simulink model "Model_of_3DOF_manipulator"  (R2023a)
settings: Solver=VariableStepAuto  StartTime=0.0  StopTime=1  RelTol=1e-3  AbsTol=1e-3
values from neighbouring files (symbols this model uses):
  K1_d = 19.4    [parameters.m]
  K1_I_xx = 9.4    [parameters.m]
  K1_I_yy = 9.4    [parameters.m]
  K1_I_zz = 0.7    [parameters.m]
  K1_K1 = 3880    [parameters.m]
  K1_K2 = 2.94    [parameters.m]
  K1_K3 = 96    [parameters.m]
  K1_K4 = 0.044    [parameters.m]
  K1_K5 = 156    [parameters.m]
  K1_l = 0.7    [parameters.m]
  K1_m = 46    [parameters.m]
  K2_d = 24.7    [parameters.m]
  K2_I_xx = 16.5    [parameters.m]
  K2_I_yy = 16.5    [parameters.m]
  K2_I_zz = 0.7    [parameters.m]
  K2_K1 = 2330    [parameters.m]
  K2_K2 = 2.8    [parameters.m]
  K2_K3 = 117    [parameters.m]
  K2_K4 = 0.043    [parameters.m]
  K2_K5 = 94    [parameters.m]
  K2_l = 0.55    [parameters.m]
  K2_m = 78    [parameters.m]
  P_d = 30.2    [parameters.m]
  P_I_xx = 33.3    [parameters.m]
  P_I_yy = 33.3    [parameters.m]
  P_I_zz = 9.1    [parameters.m]
  P_K1 = 4202    [parameters.m]
  P_K2 = 2.97    [parameters.m]
  P_K3 = 120    [parameters.m]
  P_K4 = 0.055    [parameters.m]
  P_K5 = 168    [parameters.m]
  P_l = 0.875    [parameters.m]
  P_m = 194    [parameters.m]
undefined symbols (not defined in the file or in its folder): X, Y, Z
libraries: sm_lib x21, nesl_utility x17
settings Model: Creator=ПК  LastModifiedBy=ПК
settings SolverCC: AutoScaleAbsTol=off  AlgebraicLoopSolver=TrustRegion  MaxZcPerStep=1
settings DebuggingCC: UnconnectedInputMsg=warning  UnconnectedOutputMsg=warning  UnconnectedLineMsg=warning  SymbolicDimsDataTypeCodeGenerationDiagnostic=none
settings ModelReferenceCC: EnableRefExpFcnMdlSchedulingChecks=on
settings SFSimCC: CustomCodeUndefinedFunction=UseInterfaceOnly
settings RTWCC: DLArmComputeVersion=19.05
settings SimscapeCC: SimscapeLogType=all  SimscapeLogSimulationStatistics=on  SimscapeLogDataHistory=10000

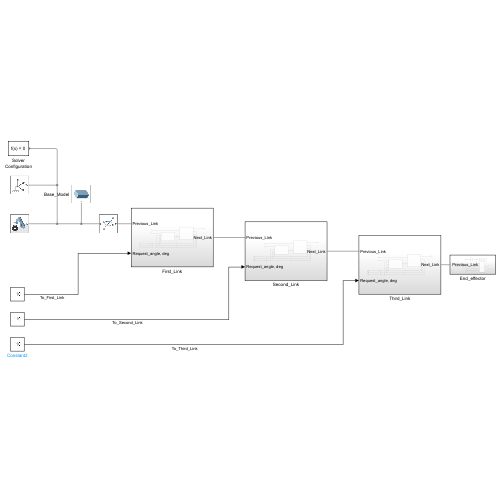
[thumbnail: Simulink's stored preview of the top-level diagram]
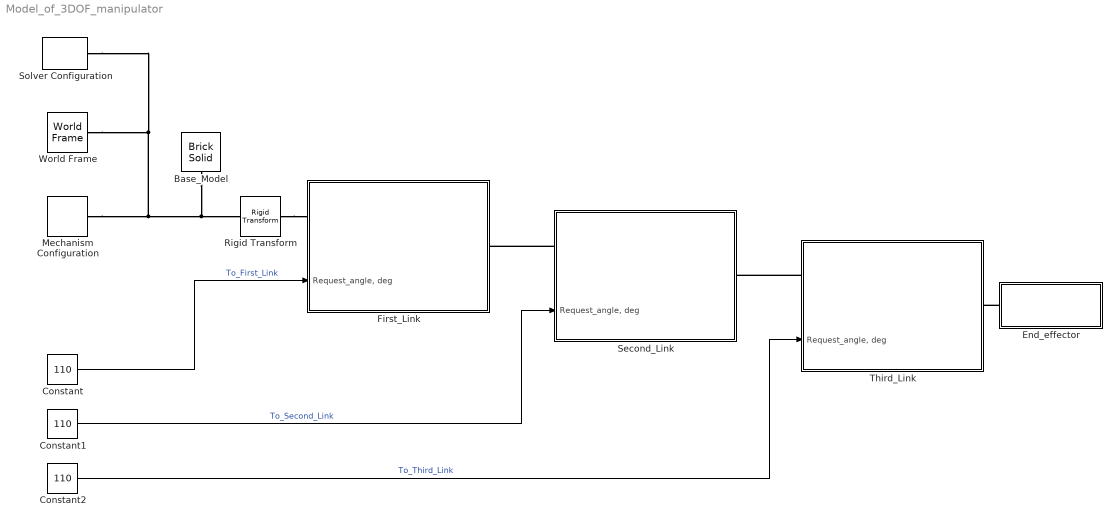
== system Model_of_3DOF_manipulator ==
  Base_Model : sm_lib/Body Elements/Brick Solid  GraphicAmbientColor=[0.15 0.15 0.15 1.0]  BasedOnType=Density  BrickDimensions=[0.5 0.5 0.5]  BrickDimensionsUnits=m  CenterOfMass=[0 0 0]  CenterOfMassUnits=m  GraphicDiffuseColor=[0.5 0.5 0.5]  Density=1000  DensityUnits=kg/m^3  DoExposeReferenceFrame=on  GraphicEmissiveColor=[0.0 0.0 0.0 1.0]  ExportEntireGeometry=off  SerializedFrames=<Frames/>  MarkerShape=Sphere  MarkerSize=10  GraphicType=FromGeometry  InertiaType=CalculateFromGeometry  Mass=1  MassUnits=kg  MomentsOfInertia=[1 1 1]  MomentsOfInertiaUnits=kg*m^2  GraphicOpacity=1.0  ProductsOfInertia=[0 0 0]  ProductsOfInertiaUnits=kg*m^2  GraphicShininess=75  GraphicSpecularColor=[0.5 0.5 0.5 1.0]  GraphicVisPropType=SimpleVisualProperties
  Constant : Constant  Value=110
  Constant1 : Constant  Value=110
  Constant2 : Constant  Value=110
  End_effector : Subsystem
  First_Link : Subsystem
      settings: PortSchema="{\"entries\":[{\"content\":{\"sides\":[{\"content\":{\"connectorIds\":[\"LConn1\",\"In1\"]},\"type\":\"ConnectorPlacement.EquallySpacedRectSide\",\"uuid\":\"66fdbe92-d6ab-4206-84fe-86206e1853da\"},{\"content\":{\"connectorIds\":[\"RConn1\"],\"side\":\"RIGHT\"},\"type\":\"ConnectorPlacement.EquallySpacedRectSide\",\"uuid\":\"85951761-cf01-4a63-8fcb-bb43d3271314\"},{\"content\":{\"side\":\"TOP\"},\"type\":\"ConnectorPlacement.EquallySpacedRectSide\",\"uuid\":\"eebc5883-fa22-4c85-b57d-f4e866a15e11\"}]},\"type\":\"ConnectorPlacement.EquallySpacedConnector\",\"uuid\":\"c98930f2-9c31-48e8-8f38-2652a55b5104\"}],\"packageUris\":[\"http://schema.mathworks.com/mf0/Connector/R2020b\"],\"version\":\"1.0\"}"
  Mechanism Configuration : sm_lib/Utilities/Mechanism Configuration  UniformGravity=Constant  GravityVector=[0 -9.80665 0]  GravityVectorUnits=m/s^2  LinearizationDelta=0.001  JointModeTransitionNonlinearIterations=2
  Rigid Transform : sm_lib/Frames and Transforms/Rigid Transform  TranslationMethod=Cartesian  TranslationStandardOffset=0  TranslationStandardOffsetUnits=m  TranslationStandardAxis=+Z  TranslationCartesianOffset=[0 0 0.25]  TranslationCartesianOffsetUnits=m  TranslationROffset=0  TranslationROffsetUnits=m  TranslationZOffset=0  TranslationZOffsetUnits=m  TranslationThetaOffset=0  TranslationThetaOffsetUnits=deg  RotationMethod=None  RotationAngleUnits=deg  RotationStandardAxis=+Z  RotationAngle=0.0  RotationArbitraryAxis=[0 0 1]  FollAlignAxisA=+X  BaseAlignAxisA=+Y  FollAlignAxisB=+Y  BaseAlignAxisB=+Z  RotationSequenceAxes=FollowerAxes  RotationSequence=XYX  RotationSequenceAngles=[0 0 0]  RotationSequenceAnglesUnits=deg  RotationMatrix=[1 0 0; 0 1 0; 0 0 1]  Quaternion=[1 0 0 0]
  Second_Link : Subsystem
      settings: PortSchema="{\"entries\":[{\"content\":{\"sides\":[{\"content\":{\"connectorIds\":[\"LConn1\",\"In1\"]},\"type\":\"ConnectorPlacement.EquallySpacedRectSide\",\"uuid\":\"66fdbe92-d6ab-4206-84fe-86206e1853da\"},{\"content\":{\"connectorIds\":[\"RConn1\"],\"side\":\"RIGHT\"},\"type\":\"ConnectorPlacement.EquallySpacedRectSide\",\"uuid\":\"85951761-cf01-4a63-8fcb-bb43d3271314\"},{\"content\":{\"side\":\"TOP\"},\"type\":\"ConnectorPlacement.EquallySpacedRectSide\",\"uuid\":\"eebc5883-fa22-4c85-b57d-f4e866a15e11\"}]},\"type\":\"ConnectorPlacement.EquallySpacedConnector\",\"uuid\":\"c98930f2-9c31-48e8-8f38-2652a55b5104\"}],\"packageUris\":[\"http://schema.mathworks.com/mf0/Connector/R2020b\"],\"version\":\"1.0\"}"
  Solver Configuration : nesl_utility/Solver Configuration  PhysicalDomain=network_engine_domain  SubClassName=solver  LeftPortType=input  RightPortType=generic  Tones=[]  Harmonics=[]  SimulateNoise=off  Profile=off  UseLocalSampling=off  EnableSwitchedLinearOptims=on  FrequencyDomain=off  UseCCode=off  RelTol=0.001  AbsTol=1e-06  MinStep=1e-09  ToWorkspace=off  RevertToSquareIcSolve=off  NumHomotopyIterations=100  PhasorMode=off  PhasorModeNumHarmonics=1  ConsistencySolver=NEWTON_XTOL_AFTER_FTOL  IndexReductionMethod=DerivativeReplacement  DoDC=off  ResidualTolerance=1e-09  ConsistencyTolSource=GLOBAL  ConsistencyAbsTol=0.001  ConsistencyRelTol=0.001  ConsistencyTolFactor=0.001  UseLocalSolver=off  LocalSolverChoice=NE_BACKWARD_EULER_ADVANCER  ResolveIndetEquations=on  FunctionEvalNumThread=1  LocalSolverSampleTime=0.001  DoFixedCost=off  MaxNonlinIter=3  MaxModeIter=2  ComputeImpulses=off  ImpulseIterations=2  LinearAlgebra=auto  LinearAlgebraNumThread=0  EquationFormulation=NE_TIME_EF  DelaysMemoryBudget=1024  AutomaticFiltering=on  FilteringTimeConstant=0.001  PartitionStorageMethod=AS_NEEDED  PartitionMemoryBudget=1024  PartitionMethod=ROBUST
  Third_Link : Subsystem
      settings: PortSchema="{\"entries\":[{\"content\":{\"sides\":[{\"content\":{\"connectorIds\":[\"LConn1\",\"In1\"]},\"type\":\"ConnectorPlacement.EquallySpacedRectSide\",\"uuid\":\"66fdbe92-d6ab-4206-84fe-86206e1853da\"},{\"content\":{\"connectorIds\":[\"RConn1\"],\"side\":\"RIGHT\"},\"type\":\"ConnectorPlacement.EquallySpacedRectSide\",\"uuid\":\"85951761-cf01-4a63-8fcb-bb43d3271314\"},{\"content\":{\"side\":\"TOP\"},\"type\":\"ConnectorPlacement.EquallySpacedRectSide\",\"uuid\":\"eebc5883-fa22-4c85-b57d-f4e866a15e11\"}]},\"type\":\"ConnectorPlacement.EquallySpacedConnector\",\"uuid\":\"c98930f2-9c31-48e8-8f38-2652a55b5104\"}],\"packageUris\":[\"http://schema.mathworks.com/mf0/Connector/R2020b\"],\"version\":\"1.0\"}"
  World Frame : sm_lib/Frames and Transforms/World Frame
  wires:
  Constant/1 -> First_Link/1("Request_angle, deg")  "To_First_Link"
  Constant1/1 -> Second_Link/1("Request_angle, deg")  "To_Second_Link"
  Constant2/1 -> Third_Link/1("Request_angle, deg")  "To_Third_Link"
  connections:
  Second_Link/LConn1 -- First_Link/RConn1
  World Frame/RConn1 -- Mechanism Configuration/RConn1 -- Rigid Transform/LConn1 -- Base_Model/RConn1 -- Solver Configuration/RConn1
  Third_Link/LConn1 -- Second_Link/RConn1
  Rigid Transform/RConn1 -- First_Link/LConn1
  End_effector/LConn1 -- Third_Link/RConn1

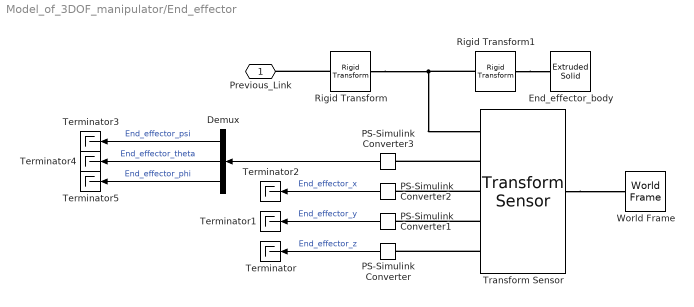
== system Model_of_3DOF_manipulator/End_effector ==
  Demux : Demux  Outputs=3
  End_effector_body : sm_lib/Body Elements/Extruded Solid  GraphicAmbientColor=[0.15 0.15 0.15 1.0]  BasedOnType=Density  CenterOfMass=[0 0 0]  CenterOfMassUnits=m  GraphicDiffuseColor=[0.5 0.5 0.5]  ExportConvexHullGeometry=off  ExtrusionCrossSection=[1 1; -1 1; -1 -1; 1 -1]  ExtrusionCrossSectionUnits=m  Density=400  DensityUnits=kg/m^3  DoExposeReferenceFrame=on  GraphicEmissiveColor=[0.0 0.0 0.0 1.0]  ExportEntireGeometry=off  ExtrusionLength=0.2  ExtrusionLengthUnits=m  ExtrusionType=Regular  SerializedFrames=<Frames/>  MarkerShape=Sphere  MarkerSize=10  GraphicType=FromGeometry  InertiaType=CalculateFromGeometry  Mass=1  MassUnits=kg  MomentsOfInertia=[1 1 1]  MomentsOfInertiaUnits=kg*m^2  PolygonNumSides=5  GraphicOpacity=1.0  PolygonOuterRadius=0.2  PolygonOuterRadiusUnits=m  ProductsOfInertia=[0 0 0]  ProductsOfInertiaUnits=kg*m^2  GraphicShininess=75  GraphicSpecularColor=[0.5 0.5 0.5 1.0]  GraphicVisPropType=SimpleVisualProperties
  PS-Simulink Converter{,1..3} (4 alike) : nesl_utility/PS-Simulink Converter  PhysicalDomain=network_engine_domain  SubClassName=ps_output  LeftPortType=input  RightPortType=output  PseudoPeriodic=off  Frequencies=[]  VectorFormat=inherit  Unit=inherit  AffineConversion=off
  Rigid Transform : sm_lib/Frames and Transforms/Rigid Transform  TranslationMethod=StandardAxis  TranslationStandardOffset=P_l  TranslationStandardOffsetUnits=m  TranslationStandardAxis=+Z  TranslationCartesianOffset=[0 0 0]  TranslationCartesianOffsetUnits=m  TranslationROffset=0  TranslationROffsetUnits=m  TranslationZOffset=0  TranslationZOffsetUnits=m  TranslationThetaOffset=0  TranslationThetaOffsetUnits=deg  RotationMethod=None  RotationAngleUnits=deg  RotationStandardAxis=+Z  RotationAngle=0.0  RotationArbitraryAxis=[0 0 1]  FollAlignAxisA=+X  BaseAlignAxisA=+Y  FollAlignAxisB=+Y  BaseAlignAxisB=+Z  RotationSequenceAxes=FollowerAxes  RotationSequence=XYX  RotationSequenceAngles=[0 0 0]  RotationSequenceAnglesUnits=deg  RotationMatrix=[1 0 0; 0 1 0; 0 0 1]  Quaternion=[1 0 0 0]
  Rigid Transform1 : sm_lib/Frames and Transforms/Rigid Transform  TranslationMethod=StandardAxis  TranslationStandardOffset=0.1  TranslationStandardOffsetUnits=m  TranslationStandardAxis=-Z  TranslationCartesianOffset=[0 0 0]  TranslationCartesianOffsetUnits=m  TranslationROffset=0  TranslationROffsetUnits=m  TranslationZOffset=0  TranslationZOffsetUnits=m  TranslationThetaOffset=0  TranslationThetaOffsetUnits=deg  RotationMethod=None  RotationAngleUnits=deg  RotationStandardAxis=+Z  RotationAngle=0.0  RotationArbitraryAxis=[0 0 1]  FollAlignAxisA=+X  BaseAlignAxisA=+Y  FollAlignAxisB=+Y  BaseAlignAxisB=+Z  RotationSequenceAxes=FollowerAxes  RotationSequence=XYX  RotationSequenceAngles=[0 0 0]  RotationSequenceAnglesUnits=deg  RotationMatrix=[1 0 0; 0 1 0; 0 0 1]  Quaternion=[1 0 0 0]
  Terminator{,1..5} (6 alike) : Terminator
  Transform Sensor : sm_lib/Frames and Transforms/Transform Sensor  MeasurementFrame=World  RotationSequence=ZXZ  SenseAngle=off  SenseAxis=off  SenseQ=off  SenseR=off  SenseRotationSequence=on  SenseOmegaX=off  SenseOmegaY=off  SenseOmegaZ=off  SenseQDot=off  SenseRDot=off  SenseRotationSequenceDot=off  SenseAlphaX=off  SenseAlphaY=off  SenseAlphaZ=off  SenseQDDot=off  SenseRDDot=off  SenseX=on  SenseY=on  SenseZ=on  SenseRad=off  SenseAzim=off  SenseDist=off  SenseInc=off  SenseXDot=off  SenseYDot=off  SenseZDot=off  SenseRadDot=off  SenseAzimDot=off  SenseDistDot=off  SenseIncDot=off  SenseXDDot=off  SenseYDDot=off  SenseZDDot=off  SenseRadDDot=off  SenseAzimDDot=off  SenseDistDDot=off  SenseIncDDot=off
  World Frame : sm_lib/Frames and Transforms/World Frame
  " Previous_Link" : PMIOPort  Side=Left
  wires:
  Demux/2 -> Terminator4/1  "End_effector_theta"
  Demux/3 -> Terminator5/1  "End_effector_phi"
  PS-Simulink Converter2/1 -> Terminator2/1  "End_effector_x"
  PS-Simulink Converter3/1 -> Demux/1
  PS-Simulink Converter/1 -> Terminator/1  "End_effector_z"
  PS-Simulink Converter1/1 -> Terminator1/1  "End_effector_y"
  Demux/1 -> Terminator3/1  "End_effector_psi"
  connections:
  Rigid Transform/LConn1 -- " Previous_Link"/RConn1
  Rigid Transform1/LConn1 -- End_effector_body/RConn1
  Transform Sensor/LConn1 -- World Frame/RConn1
  Rigid Transform/RConn1 -- Rigid Transform1/RConn1 -- Transform Sensor/RConn1
  Transform Sensor/RConn2 -- PS-Simulink Converter3/LConn1
  Transform Sensor/RConn4 -- PS-Simulink Converter1/LConn1
  Transform Sensor/RConn3 -- PS-Simulink Converter2/LConn1
  Transform Sensor/RConn5 -- PS-Simulink Converter/LConn1

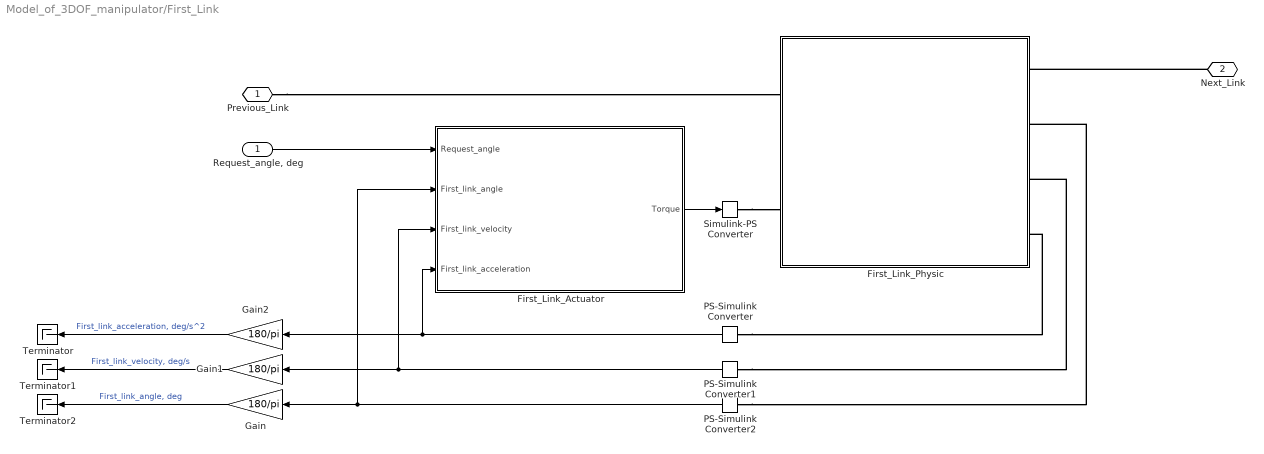
== system Model_of_3DOF_manipulator/First_Link ==
  "Request_angle, deg" : Inport
  First_Link_Actuator : Subsystem
  First_Link_Physic : Subsystem
  Gain : Gain  Gain=180/pi
  Gain1 : Gain  Gain=180/pi
  Gain2 : Gain  Gain=180/pi
  PS-Simulink Converter : nesl_utility/PS-Simulink Converter  PhysicalDomain=network_engine_domain  SubClassName=ps_output  LeftPortType=input  RightPortType=output  PseudoPeriodic=off  Frequencies=[]  VectorFormat=inherit  Unit=inherit  AffineConversion=off
  PS-Simulink Converter1 : nesl_utility/PS-Simulink Converter  PhysicalDomain=network_engine_domain  SubClassName=ps_output  LeftPortType=input  RightPortType=output  PseudoPeriodic=off  Frequencies=[]  VectorFormat=inherit  Unit=inherit  AffineConversion=off
  PS-Simulink Converter2 : nesl_utility/PS-Simulink Converter  PhysicalDomain=network_engine_domain  SubClassName=ps_output  LeftPortType=input  RightPortType=output  PseudoPeriodic=off  Frequencies=[]  VectorFormat=inherit  Unit=inherit  AffineConversion=off
  Simulink-PS Converter : nesl_utility/Simulink-PS Converter  PhysicalDomain=network_engine_domain  SubClassName=ps_input  LeftPortType=input  RightPortType=output  PseudoPeriodic=off  Frequencies=[]  NoiseDistribution=none  NoiseParameters=[]  Unit=1  AffineConversion=off  FilteringAndDerivatives=provide  SimscapeFilterOrder=1  InputFilterTimeConstant=0.001  UdotUserProvided=0
  Terminator : Terminator
  Terminator1 : Terminator
  Terminator2 : Terminator
  Previous_Link : PMIOPort  Side=Left
  Next_Link : PMIOPort  Port=2  Side=Right
  wires:
  First_Link_Actuator/1(Torque) -> Simulink-PS Converter/1
  PS-Simulink Converter/1 -> First_Link_Actuator/4(First_link_acceleration), Gain2/1
  PS-Simulink Converter1/1 -> First_Link_Actuator/3(First_link_velocity), Gain1/1
  PS-Simulink Converter2/1 -> Gain/1, First_Link_Actuator/2(First_link_angle)
  "Request_angle, deg"/1 -> First_Link_Actuator/1(Request_angle)
  Gain2/1 -> Terminator/1  "First_link_acceleration, deg/s^2"
  Gain/1 -> Terminator2/1  "First_link_angle, deg"
  Gain1/1 -> Terminator1/1  "First_link_velocity, deg/s"
  connections:
  Simulink-PS Converter/RConn1 -- First_Link_Physic/LConn2
  PS-Simulink Converter/LConn1 -- First_Link_Physic/RConn4
  PS-Simulink Converter1/LConn1 -- First_Link_Physic/RConn3
  PS-Simulink Converter2/LConn1 -- First_Link_Physic/RConn2
  Next_Link/RConn1 -- First_Link_Physic/RConn1
  Previous_Link/RConn1 -- First_Link_Physic/LConn1

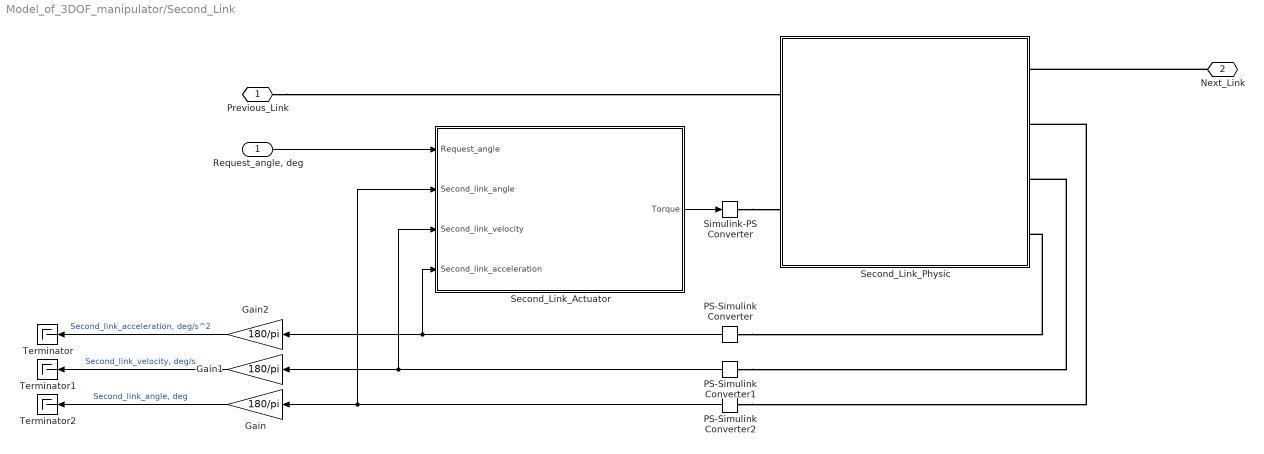
== system Model_of_3DOF_manipulator/Second_Link ==
  "Request_angle, deg" : Inport
  Gain : Gain  Gain=180/pi
  Gain1 : Gain  Gain=180/pi
  Gain2 : Gain  Gain=180/pi
  PS-Simulink Converter : nesl_utility/PS-Simulink Converter  PhysicalDomain=network_engine_domain  SubClassName=ps_output  LeftPortType=input  RightPortType=output  PseudoPeriodic=off  Frequencies=[]  VectorFormat=inherit  Unit=inherit  AffineConversion=off
  PS-Simulink Converter1 : nesl_utility/PS-Simulink Converter  PhysicalDomain=network_engine_domain  SubClassName=ps_output  LeftPortType=input  RightPortType=output  PseudoPeriodic=off  Frequencies=[]  VectorFormat=inherit  Unit=inherit  AffineConversion=off
  PS-Simulink Converter2 : nesl_utility/PS-Simulink Converter  PhysicalDomain=network_engine_domain  SubClassName=ps_output  LeftPortType=input  RightPortType=output  PseudoPeriodic=off  Frequencies=[]  VectorFormat=inherit  Unit=inherit  AffineConversion=off
  Second_Link_Actuator : Subsystem
  Second_Link_Physic : Subsystem
  Simulink-PS Converter : nesl_utility/Simulink-PS Converter  PhysicalDomain=network_engine_domain  SubClassName=ps_input  LeftPortType=input  RightPortType=output  PseudoPeriodic=off  Frequencies=[]  NoiseDistribution=none  NoiseParameters=[]  Unit=1  AffineConversion=off  FilteringAndDerivatives=provide  SimscapeFilterOrder=1  InputFilterTimeConstant=0.001  UdotUserProvided=0
  Terminator : Terminator
  Terminator1 : Terminator
  Terminator2 : Terminator
  Previous_Link : PMIOPort  Side=Left
  Next_Link : PMIOPort  Port=2  Side=Right
  wires:
  Second_Link_Actuator/1(Torque) -> Simulink-PS Converter/1
  PS-Simulink Converter/1 -> Second_Link_Actuator/4(Second_link_acceleration), Gain2/1
  PS-Simulink Converter1/1 -> Second_Link_Actuator/3(Second_link_velocity), Gain1/1
  PS-Simulink Converter2/1 -> Gain/1, Second_Link_Actuator/2(Second_link_angle)
  "Request_angle, deg"/1 -> Second_Link_Actuator/1(Request_angle)
  Gain2/1 -> Terminator/1  "Second_link_acceleration, deg/s^2"
  Gain/1 -> Terminator2/1  "Second_link_angle, deg"
  Gain1/1 -> Terminator1/1  "Second_link_velocity, deg/s"
  connections:
  Simulink-PS Converter/RConn1 -- Second_Link_Physic/LConn2
  PS-Simulink Converter/LConn1 -- Second_Link_Physic/RConn4
  PS-Simulink Converter1/LConn1 -- Second_Link_Physic/RConn3
  PS-Simulink Converter2/LConn1 -- Second_Link_Physic/RConn2
  Next_Link/RConn1 -- Second_Link_Physic/RConn1
  Previous_Link/RConn1 -- Second_Link_Physic/LConn1

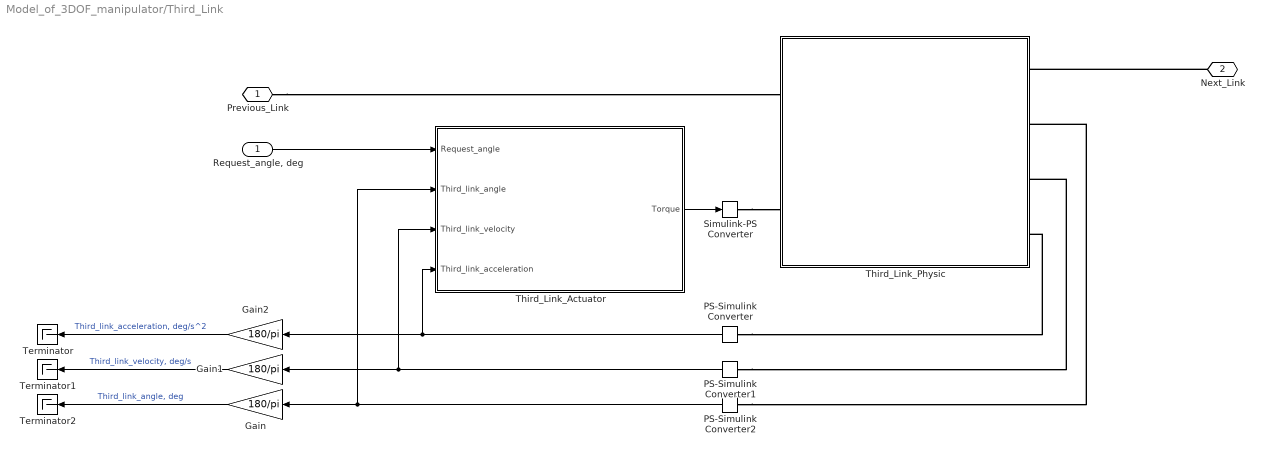
== system Model_of_3DOF_manipulator/Third_Link ==
  "Request_angle, deg" : Inport
  Gain : Gain  Gain=180/pi
  Gain1 : Gain  Gain=180/pi
  Gain2 : Gain  Gain=180/pi
  PS-Simulink Converter : nesl_utility/PS-Simulink Converter  PhysicalDomain=network_engine_domain  SubClassName=ps_output  LeftPortType=input  RightPortType=output  PseudoPeriodic=off  Frequencies=[]  VectorFormat=inherit  Unit=inherit  AffineConversion=off
  PS-Simulink Converter1 : nesl_utility/PS-Simulink Converter  PhysicalDomain=network_engine_domain  SubClassName=ps_output  LeftPortType=input  RightPortType=output  PseudoPeriodic=off  Frequencies=[]  VectorFormat=inherit  Unit=inherit  AffineConversion=off
  PS-Simulink Converter2 : nesl_utility/PS-Simulink Converter  PhysicalDomain=network_engine_domain  SubClassName=ps_output  LeftPortType=input  RightPortType=output  PseudoPeriodic=off  Frequencies=[]  VectorFormat=inherit  Unit=inherit  AffineConversion=off
  Simulink-PS Converter : nesl_utility/Simulink-PS Converter  PhysicalDomain=network_engine_domain  SubClassName=ps_input  LeftPortType=input  RightPortType=output  PseudoPeriodic=off  Frequencies=[]  NoiseDistribution=none  NoiseParameters=[]  Unit=1  AffineConversion=off  FilteringAndDerivatives=provide  SimscapeFilterOrder=1  InputFilterTimeConstant=0.001  UdotUserProvided=0
  Terminator : Terminator
  Terminator1 : Terminator
  Terminator2 : Terminator
  Third_Link_Actuator : Subsystem
  Third_Link_Physic : Subsystem
  Previous_Link : PMIOPort  Side=Left
  Next_Link : PMIOPort  Port=2  Side=Right
  wires:
  Third_Link_Actuator/1(Torque) -> Simulink-PS Converter/1
  PS-Simulink Converter/1 -> Third_Link_Actuator/4(Third_link_acceleration), Gain2/1
  PS-Simulink Converter1/1 -> Third_Link_Actuator/3(Third_link_velocity), Gain1/1
  PS-Simulink Converter2/1 -> Gain/1, Third_Link_Actuator/2(Third_link_angle)
  "Request_angle, deg"/1 -> Third_Link_Actuator/1(Request_angle)
  Gain2/1 -> Terminator/1  "Third_link_acceleration, deg/s^2"
  Gain/1 -> Terminator2/1  "Third_link_angle, deg"
  Gain1/1 -> Terminator1/1  "Third_link_velocity, deg/s"
  connections:
  Simulink-PS Converter/RConn1 -- Third_Link_Physic/LConn2
  PS-Simulink Converter/LConn1 -- Third_Link_Physic/RConn4
  PS-Simulink Converter1/LConn1 -- Third_Link_Physic/RConn3
  PS-Simulink Converter2/LConn1 -- Third_Link_Physic/RConn2
  Next_Link/RConn1 -- Third_Link_Physic/RConn1
  Previous_Link/RConn1 -- Third_Link_Physic/LConn1

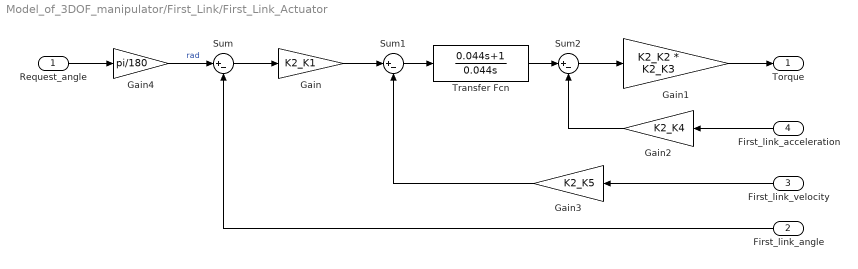
== system Model_of_3DOF_manipulator/First_Link/First_Link_Actuator ==
  Request_angle : Inport
  First_link_angle : Inport  Port=2
  First_link_velocity : Inport  Port=3
  First_link_acceleration : Inport  Port=4
  Gain : Gain  Gain=K2_K1
  Gain1 : Gain  Gain=K2_K2 * K2_K3
  Gain2 : Gain  Gain=K2_K4
  Gain3 : Gain  Gain=K2_K5
  Gain4 : Gain  Gain=pi/180
  Sum : Sum  Inputs=|+-
  Sum1 : Sum  Inputs=|+-
  Sum2 : Sum  Inputs=|+-
  Transfer Fcn : TransferFcn  Numerator=[0.044 1]  Denominator=[0.044 0]
  Torque : Outport
  wires:
  Request_angle/1 -> Gain4/1
  Sum/1 -> Gain/1
  Gain/1 -> Sum1/1
  Sum1/1 -> Transfer Fcn/1
  Transfer Fcn/1 -> Sum2/1
  Sum2/1 -> Gain1/1
  Gain1/1 -> Torque/1
  First_link_velocity/1 -> Gain3/1
  First_link_acceleration/1 -> Gain2/1
  Gain2/1 -> Sum2/2
  Gain3/1 -> Sum1/2
  First_link_angle/1 -> Sum/2
  Gain4/1 -> Sum/1  "rad"

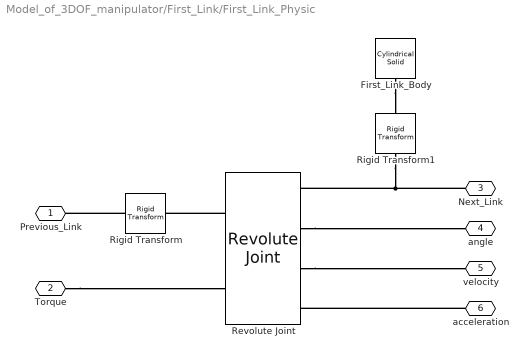
== system Model_of_3DOF_manipulator/First_Link/First_Link_Physic ==
  First_Link_Body : sm_lib/Body Elements/Cylindrical Solid  GraphicAmbientColor=[0.15 0.15 0.15 1.0]  BasedOnType=Density  CenterOfMass=[0 0 0]  CenterOfMassUnits=m  GraphicDiffuseColor=[0.5 0.5 0.5]  CylinderLength=K2_l  CylinderLengthUnits=m  CylinderRadius=K2_d/2  CylinderRadiusUnits=cm  Density=1000  DensityUnits=kg/m^3  DoExposeReferenceFrame=on  GraphicEmissiveColor=[0.0 0.0 0.0 1.0]  ExportEntireGeometry=off  SerializedFrames=<Frames/>  MarkerShape=Sphere  MarkerSize=10  GraphicType=FromGeometry  InertiaType=Custom  Mass=K2_m  MassUnits=kg  MomentsOfInertia=[K2_I_xx K2_I_yy K2_I_zz]  MomentsOfInertiaUnits=kg*m^2  GraphicOpacity=1.0  ProductsOfInertia=[0 0 0]  ProductsOfInertiaUnits=kg*m^2  GraphicShininess=75  GraphicSpecularColor=[0.5 0.5 0.5 1.0]  GraphicVisPropType=SimpleVisualProperties
  Revolute Joint : sm_lib/Joints/Revolute Joint  JointMode=Normal  SenseConstraintForce=off  SenseConstraintForceX=off  SenseConstraintForceY=off  SenseConstraintForceZ=off  SenseConstraintTorque=off  SenseConstraintTorqueX=off  SenseConstraintTorqueY=off  SenseConstraintTorqueZ=off  SenseTotalForce=off  SenseTotalForceX=off  SenseTotalForceY=off  SenseTotalForceZ=off  SenseTotalTorque=off  SenseTotalTorqueX=off  SenseTotalTorqueY=off  SenseTotalTorqueZ=off  CompositeWrenchDir=FollowerOnBase  CompositeWrenchFrame=BaseFrame  EquilibriumPosition=0  EquilibriumPositionUnits=deg  SpringStiffness=0  SpringStiffnessUnits=N*m/deg  DampingCoefficient=0  DampingCoefficientUnits=N*m/(deg/s)  TorqueActuationMode=InputTorque  MotionActuationMode=ComputedMotion  SensePosition=on  SenseVelocity=on  SenseAcceleration=on  SenseTorqueForce=off  SenseLowerLimitTorqueForce=off  SenseUpperLimitTorqueForce=off  LowerLimitSpecify=on  LowerLimitBound=-100  LowerLimitBoundUnits=deg  LowerLimitStiffness=1e6  LowerLimitStiffnessUnits=N*m/deg  LowerLimitDamping=100  LowerLimitDampingUnits=N*m/(deg/s)  LowerLimitTransitionRegionWidth=0.1  LowerLimitTransitionRegionWidthUnits=deg  UpperLimitSpecify=on  UpperLimitBound=100  UpperLimitBoundUnits=deg  UpperLimitStiffness=1e6  UpperLimitStiffnessUnits=N*m/deg  UpperLimitDamping=100  UpperLimitDampingUnits=N*m/(deg/s)  UpperLimitTransitionRegionWidth=0.1  UpperLimitTransitionRegionWidthUnits=deg  PositionTargetSpecify=off  PositionTargetPriority=High  PositionTargetValue=0  PositionTargetValueUnits=deg  VelocityTargetSpecify=off  VelocityTargetPriority=High  VelocityTargetValue=0  VelocityTargetValueUnits=deg/s
  Rigid Transform : sm_lib/Frames and Transforms/Rigid Transform  TranslationMethod=None  TranslationStandardOffset=K2_l/2  TranslationStandardOffsetUnits=m  TranslationStandardAxis=+Z  TranslationCartesianOffset=[0 0 0]  TranslationCartesianOffsetUnits=m  TranslationROffset=0  TranslationROffsetUnits=m  TranslationZOffset=0  TranslationZOffsetUnits=m  TranslationThetaOffset=0  TranslationThetaOffsetUnits=deg  RotationMethod=StandardAxis  RotationAngleUnits=deg  RotationStandardAxis=+X  RotationAngle=90  RotationArbitraryAxis=[0 0 1]  FollAlignAxisA=+X  BaseAlignAxisA=+Y  FollAlignAxisB=+Y  BaseAlignAxisB=+Z  RotationSequenceAxes=FollowerAxes  RotationSequence=XYX  RotationSequenceAngles=[0 0 0]  RotationSequenceAnglesUnits=deg  RotationMatrix=[1 0 0; 0 1 0; 0 0 1]  Quaternion=[1 0 0 0]
  Rigid Transform1 : sm_lib/Frames and Transforms/Rigid Transform  TranslationMethod=StandardAxis  TranslationStandardOffset=K2_l/2  TranslationStandardOffsetUnits=m  TranslationStandardAxis=-Z  TranslationCartesianOffset=[0 0 0]  TranslationCartesianOffsetUnits=m  TranslationROffset=0  TranslationROffsetUnits=m  TranslationZOffset=0  TranslationZOffsetUnits=m  TranslationThetaOffset=0  TranslationThetaOffsetUnits=deg  RotationMethod=StandardAxis  RotationAngleUnits=deg  RotationStandardAxis=+X  RotationAngle=90  RotationArbitraryAxis=[0 0 1]  FollAlignAxisA=+X  BaseAlignAxisA=+Y  FollAlignAxisB=+Y  BaseAlignAxisB=+Z  RotationSequenceAxes=FollowerAxes  RotationSequence=XYX  RotationSequenceAngles=[0 0 0]  RotationSequenceAnglesUnits=deg  RotationMatrix=[1 0 0; 0 1 0; 0 0 1]  Quaternion=[1 0 0 0]
  Previous_Link : PMIOPort  Side=Left
  Torque : PMIOPort  Port=2  Side=Left
  Next_Link : PMIOPort  Port=3  Side=Right
  angle : PMIOPort  Port=4  Side=Right
  velocity : PMIOPort  Port=5  Side=Right
  acceleration : PMIOPort  Port=6  Side=Right
  connections:
  Rigid Transform/LConn1 -- Previous_Link/RConn1
  Revolute Joint/LConn1 -- Rigid Transform/RConn1
  Torque/RConn1 -- Revolute Joint/LConn2
  Revolute Joint/RConn2 -- angle/RConn1
  acceleration/RConn1 -- Revolute Joint/RConn4
  Revolute Joint/RConn3 -- velocity/RConn1
  First_Link_Body/RConn1 -- Rigid Transform1/LConn1
  Rigid Transform1/RConn1 -- Next_Link/RConn1 -- Revolute Joint/RConn1

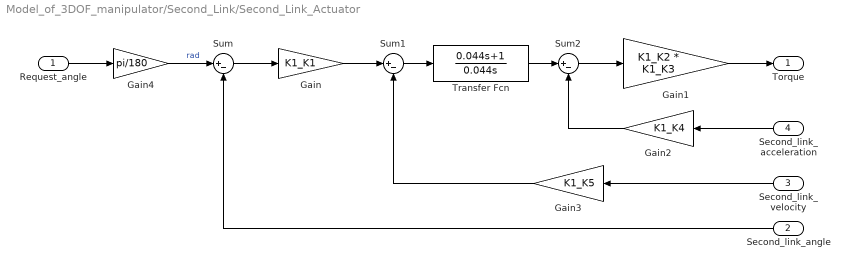
== system Model_of_3DOF_manipulator/Second_Link/Second_Link_Actuator ==
  Request_angle : Inport
  Second_link_angle : Inport  Port=2
  Second_link_velocity : Inport  Port=3
  Second_link_acceleration : Inport  Port=4
  Gain : Gain  Gain=K1_K1
  Gain1 : Gain  Gain=K1_K2 * K1_K3
  Gain2 : Gain  Gain=K1_K4
  Gain3 : Gain  Gain=K1_K5
  Gain4 : Gain  Gain=pi/180
  Sum : Sum  Inputs=|+-
  Sum1 : Sum  Inputs=|+-
  Sum2 : Sum  Inputs=|+-
  Transfer Fcn : TransferFcn  Numerator=[0.044 1]  Denominator=[0.044 0]
  Torque : Outport
  wires:
  Request_angle/1 -> Gain4/1
  Sum/1 -> Gain/1
  Gain/1 -> Sum1/1
  Sum1/1 -> Transfer Fcn/1
  Transfer Fcn/1 -> Sum2/1
  Sum2/1 -> Gain1/1
  Gain1/1 -> Torque/1
  Second_link_velocity/1 -> Gain3/1
  Second_link_acceleration/1 -> Gain2/1
  Gain2/1 -> Sum2/2
  Gain3/1 -> Sum1/2
  Second_link_angle/1 -> Sum/2
  Gain4/1 -> Sum/1  "rad"

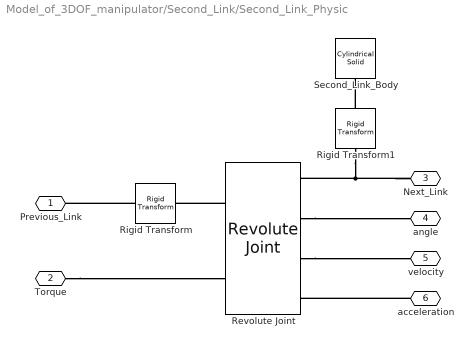
== system Model_of_3DOF_manipulator/Second_Link/Second_Link_Physic ==
  Revolute Joint : sm_lib/Joints/Revolute Joint  JointMode=Normal  SenseConstraintForce=off  SenseConstraintForceX=off  SenseConstraintForceY=off  SenseConstraintForceZ=off  SenseConstraintTorque=off  SenseConstraintTorqueX=off  SenseConstraintTorqueY=off  SenseConstraintTorqueZ=off  SenseTotalForce=off  SenseTotalForceX=off  SenseTotalForceY=off  SenseTotalForceZ=off  SenseTotalTorque=off  SenseTotalTorqueX=off  SenseTotalTorqueY=off  SenseTotalTorqueZ=off  CompositeWrenchDir=FollowerOnBase  CompositeWrenchFrame=BaseFrame  EquilibriumPosition=0  EquilibriumPositionUnits=deg  SpringStiffness=0  SpringStiffnessUnits=N*m/deg  DampingCoefficient=0  DampingCoefficientUnits=N*m/(deg/s)  TorqueActuationMode=InputTorque  MotionActuationMode=ComputedMotion  SensePosition=on  SenseVelocity=on  SenseAcceleration=on  SenseTorqueForce=off  SenseLowerLimitTorqueForce=off  SenseUpperLimitTorqueForce=off  LowerLimitSpecify=on  LowerLimitBound=-105  LowerLimitBoundUnits=deg  LowerLimitStiffness=1e6  LowerLimitStiffnessUnits=N*m/deg  LowerLimitDamping=10  LowerLimitDampingUnits=N*m/(deg/s)  LowerLimitTransitionRegionWidth=0.1  LowerLimitTransitionRegionWidthUnits=deg  UpperLimitSpecify=on  UpperLimitBound=105  UpperLimitBoundUnits=deg  UpperLimitStiffness=1e6  UpperLimitStiffnessUnits=N*m/deg  UpperLimitDamping=10  UpperLimitDampingUnits=N*m/(deg/s)  UpperLimitTransitionRegionWidth=0.1  UpperLimitTransitionRegionWidthUnits=deg  PositionTargetSpecify=off  PositionTargetPriority=High  PositionTargetValue=0  PositionTargetValueUnits=deg  VelocityTargetSpecify=off  VelocityTargetPriority=High  VelocityTargetValue=0  VelocityTargetValueUnits=deg/s
  Rigid Transform : sm_lib/Frames and Transforms/Rigid Transform  TranslationMethod=StandardAxis  TranslationStandardOffset=K2_l  TranslationStandardOffsetUnits=m  TranslationStandardAxis=+Y  TranslationCartesianOffset=[-K2_l 0 0]  TranslationCartesianOffsetUnits=m  TranslationROffset=0  TranslationROffsetUnits=m  TranslationZOffset=0  TranslationZOffsetUnits=m  TranslationThetaOffset=0  TranslationThetaOffsetUnits=deg  RotationMethod=None  RotationAngleUnits=deg  RotationStandardAxis=+Y  RotationAngle=90  RotationArbitraryAxis=[0 0 1]  FollAlignAxisA=+X  BaseAlignAxisA=+Y  FollAlignAxisB=+Y  BaseAlignAxisB=+Z  RotationSequenceAxes=FollowerAxes  RotationSequence=XYX  RotationSequenceAngles=[0 0 0]  RotationSequenceAnglesUnits=deg  RotationMatrix=[1 0 0; 0 1 0; 0 0 1]  Quaternion=[1 0 0 0]
  Rigid Transform1 : sm_lib/Frames and Transforms/Rigid Transform  TranslationMethod=StandardAxis  TranslationStandardOffset=K1_l/2  TranslationStandardOffsetUnits=m  TranslationStandardAxis=-Z  TranslationCartesianOffset=[-K2_l 0 0]  TranslationCartesianOffsetUnits=m  TranslationROffset=0  TranslationROffsetUnits=m  TranslationZOffset=0  TranslationZOffsetUnits=m  TranslationThetaOffset=0  TranslationThetaOffsetUnits=deg  RotationMethod=StandardAxis  RotationAngleUnits=deg  RotationStandardAxis=-Y  RotationAngle=90  RotationArbitraryAxis=[0 0 1]  FollAlignAxisA=+X  BaseAlignAxisA=+Y  FollAlignAxisB=+Y  BaseAlignAxisB=+Z  RotationSequenceAxes=FollowerAxes  RotationSequence=XYX  RotationSequenceAngles=[0 0 0]  RotationSequenceAnglesUnits=deg  RotationMatrix=[1 0 0; 0 1 0; 0 0 1]  Quaternion=[1 0 0 0]
  Second_Link_Body : sm_lib/Body Elements/Cylindrical Solid  GraphicAmbientColor=[0.15 0.15 0.15 1.0]  BasedOnType=Density  CenterOfMass=[0 0 0]  CenterOfMassUnits=m  GraphicDiffuseColor=[0.5 0.5 0.5]  CylinderLength=K1_l  CylinderLengthUnits=m  CylinderRadius=K1_d/2  CylinderRadiusUnits=cm  Density=1000  DensityUnits=kg/m^3  DoExposeReferenceFrame=on  GraphicEmissiveColor=[0.0 0.0 0.0 1.0]  ExportEntireGeometry=off  SerializedFrames=<Frames/>  MarkerShape=Sphere  MarkerSize=10  GraphicType=FromGeometry  InertiaType=Custom  Mass=K1_m  MassUnits=kg  MomentsOfInertia=[K1_I_xx K1_I_yy K1_I_zz]  MomentsOfInertiaUnits=kg*m^2  GraphicOpacity=1.0  ProductsOfInertia=[0 0 0]  ProductsOfInertiaUnits=kg*m^2  GraphicShininess=75  GraphicSpecularColor=[0.5 0.5 0.5 1.0]  GraphicVisPropType=SimpleVisualProperties
  Previous_Link : PMIOPort  Side=Left
  Torque : PMIOPort  Port=2  Side=Left
  Next_Link : PMIOPort  Port=3  Side=Right
  angle : PMIOPort  Port=4  Side=Right
  velocity : PMIOPort  Port=5  Side=Right
  acceleration : PMIOPort  Port=6  Side=Right
  connections:
  Rigid Transform/LConn1 -- Previous_Link/RConn1
  Revolute Joint/LConn1 -- Rigid Transform/RConn1
  Torque/RConn1 -- Revolute Joint/LConn2
  Revolute Joint/RConn2 -- angle/RConn1
  Next_Link/RConn1 -- Rigid Transform1/RConn1 -- Revolute Joint/RConn1
  acceleration/RConn1 -- Revolute Joint/RConn4
  Revolute Joint/RConn3 -- velocity/RConn1
  Rigid Transform1/LConn1 -- Second_Link_Body/RConn1

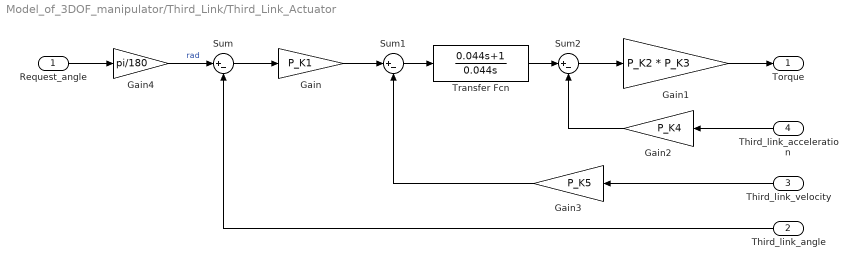
== system Model_of_3DOF_manipulator/Third_Link/Third_Link_Actuator ==
  Request_angle : Inport
  Third_link_angle : Inport  Port=2
  Third_link_velocity : Inport  Port=3
  Third_link_acceleration : Inport  Port=4
  Gain : Gain  Gain=P_K1
  Gain1 : Gain  Gain=P_K2 * P_K3
  Gain2 : Gain  Gain=P_K4
  Gain3 : Gain  Gain=P_K5
  Gain4 : Gain  Gain=pi/180
  Sum : Sum  Inputs=|+-
  Sum1 : Sum  Inputs=|+-
  Sum2 : Sum  Inputs=|+-
  Transfer Fcn : TransferFcn  Numerator=[0.044 1]  Denominator=[0.044 0]
  Torque : Outport
  wires:
  Request_angle/1 -> Gain4/1
  Sum/1 -> Gain/1
  Gain/1 -> Sum1/1
  Sum1/1 -> Transfer Fcn/1
  Transfer Fcn/1 -> Sum2/1
  Sum2/1 -> Gain1/1
  Gain1/1 -> Torque/1
  Third_link_velocity/1 -> Gain3/1
  Third_link_acceleration/1 -> Gain2/1
  Gain2/1 -> Sum2/2
  Gain3/1 -> Sum1/2
  Third_link_angle/1 -> Sum/2
  Gain4/1 -> Sum/1  "rad"

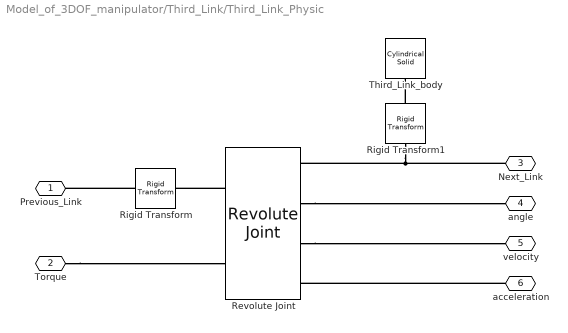
== system Model_of_3DOF_manipulator/Third_Link/Third_Link_Physic ==
  Revolute Joint : sm_lib/Joints/Revolute Joint  JointMode=Normal  SenseConstraintForce=off  SenseConstraintForceX=off  SenseConstraintForceY=off  SenseConstraintForceZ=off  SenseConstraintTorque=off  SenseConstraintTorqueX=off  SenseConstraintTorqueY=off  SenseConstraintTorqueZ=off  SenseTotalForce=off  SenseTotalForceX=off  SenseTotalForceY=off  SenseTotalForceZ=off  SenseTotalTorque=off  SenseTotalTorqueX=off  SenseTotalTorqueY=off  SenseTotalTorqueZ=off  CompositeWrenchDir=FollowerOnBase  CompositeWrenchFrame=BaseFrame  EquilibriumPosition=0  EquilibriumPositionUnits=deg  SpringStiffness=0  SpringStiffnessUnits=N*m/deg  DampingCoefficient=0  DampingCoefficientUnits=N*m/(deg/s)  TorqueActuationMode=InputTorque  MotionActuationMode=ComputedMotion  SensePosition=on  SenseVelocity=on  SenseAcceleration=on  SenseTorqueForce=off  SenseLowerLimitTorqueForce=off  SenseUpperLimitTorqueForce=off  LowerLimitSpecify=off  LowerLimitBound=-90  LowerLimitBoundUnits=deg  LowerLimitStiffness=1e4  LowerLimitStiffnessUnits=N*m/deg  LowerLimitDamping=10  LowerLimitDampingUnits=N*m/(deg/s)  LowerLimitTransitionRegionWidth=0.1  LowerLimitTransitionRegionWidthUnits=deg  UpperLimitSpecify=off  UpperLimitBound=90  UpperLimitBoundUnits=deg  UpperLimitStiffness=1e4  UpperLimitStiffnessUnits=N*m/deg  UpperLimitDamping=10  UpperLimitDampingUnits=N*m/(deg/s)  UpperLimitTransitionRegionWidth=0.1  UpperLimitTransitionRegionWidthUnits=deg  PositionTargetSpecify=off  PositionTargetPriority=High  PositionTargetValue=0  PositionTargetValueUnits=deg  VelocityTargetSpecify=off  VelocityTargetPriority=High  VelocityTargetValue=0  VelocityTargetValueUnits=deg/s
  Rigid Transform : sm_lib/Frames and Transforms/Rigid Transform  TranslationMethod=StandardAxis  TranslationStandardOffset=K1_l  TranslationStandardOffsetUnits=m  TranslationStandardAxis=+X  TranslationCartesianOffset=[0 0 0]  TranslationCartesianOffsetUnits=m  TranslationROffset=0  TranslationROffsetUnits=m  TranslationZOffset=0  TranslationZOffsetUnits=m  TranslationThetaOffset=0  TranslationThetaOffsetUnits=deg  RotationMethod=StandardAxis  RotationAngleUnits=deg  RotationStandardAxis=-Y  RotationAngle=-90  RotationArbitraryAxis=[0 0 1]  FollAlignAxisA=+X  BaseAlignAxisA=+Y  FollAlignAxisB=+Y  BaseAlignAxisB=+Z  RotationSequenceAxes=FollowerAxes  RotationSequence=XYX  RotationSequenceAngles=[0 0 0]  RotationSequenceAnglesUnits=deg  RotationMatrix=[1 0 0; 0 1 0; 0 0 1]  Quaternion=[1 0 0 0]
  Rigid Transform1 : sm_lib/Frames and Transforms/Rigid Transform  TranslationMethod=StandardAxis  TranslationStandardOffset=P_l/2  TranslationStandardOffsetUnits=m  TranslationStandardAxis=-Z  TranslationCartesianOffset=[0 0 0]  TranslationCartesianOffsetUnits=m  TranslationROffset=0  TranslationROffsetUnits=m  TranslationZOffset=0  TranslationZOffsetUnits=m  TranslationThetaOffset=0  TranslationThetaOffsetUnits=deg  RotationMethod=None  RotationAngleUnits=deg  RotationStandardAxis=+Z  RotationAngle=-90  RotationArbitraryAxis=[0 0 1]  FollAlignAxisA=+X  BaseAlignAxisA=+Y  FollAlignAxisB=+Y  BaseAlignAxisB=+Z  RotationSequenceAxes=FollowerAxes  RotationSequence=XYX  RotationSequenceAngles=[0 0 0]  RotationSequenceAnglesUnits=deg  RotationMatrix=[1 0 0; 0 1 0; 0 0 1]  Quaternion=[1 0 0 0]
  Third_Link_body : sm_lib/Body Elements/Cylindrical Solid  GraphicAmbientColor=[0.15 0.15 0.15 1.0]  BasedOnType=Density  CenterOfMass=[0 0 0]  CenterOfMassUnits=m  GraphicDiffuseColor=[0.5 0.5 0.5]  CylinderLength=P_l  CylinderLengthUnits=m  CylinderRadius=P_d/2  CylinderRadiusUnits=cm  Density=1000  DensityUnits=kg/m^3  DoExposeReferenceFrame=on  GraphicEmissiveColor=[0.0 0.0 0.0 1.0]  ExportEntireGeometry=off  SerializedFrames=<Frames/>  MarkerShape=Sphere  MarkerSize=10  GraphicType=FromGeometry  InertiaType=Custom  Mass=P_m  MassUnits=kg  MomentsOfInertia=[P_I_xx P_I_yy P_I_zz]  MomentsOfInertiaUnits=kg*m^2  GraphicOpacity=1.0  ProductsOfInertia=[0 0 0]  ProductsOfInertiaUnits=kg*m^2  GraphicShininess=75  GraphicSpecularColor=[0.5 0.5 0.5 1.0]  GraphicVisPropType=SimpleVisualProperties
  Previous_Link : PMIOPort  Side=Left
  Torque : PMIOPort  Port=2  Side=Left
  Next_Link : PMIOPort  Port=3  Side=Right
  angle : PMIOPort  Port=4  Side=Right
  velocity : PMIOPort  Port=5  Side=Right
  acceleration : PMIOPort  Port=6  Side=Right
  connections:
  Rigid Transform/LConn1 -- Previous_Link/RConn1
  Revolute Joint/LConn1 -- Rigid Transform/RConn1
  Torque/RConn1 -- Revolute Joint/LConn2
  Revolute Joint/RConn2 -- angle/RConn1
  Next_Link/RConn1 -- Rigid Transform1/RConn1 -- Revolute Joint/RConn1
  acceleration/RConn1 -- Revolute Joint/RConn4
  Revolute Joint/RConn3 -- velocity/RConn1
  Rigid Transform1/LConn1 -- Third_Link_body/RConn1
